simulink model "ControlDataSSM0709"  (R2023b)
settings: Solver=FixedStepAuto  StartTime=0.0  StopTime=inf  FixedStep=0.01  RelTol=1e-3
undefined symbols (not defined in the file): Down, Pull
libraries: simulink x39, speedgoatlib_IO691 x23, canmsglib x22, slrealtimeutilitieslib x1, slrealtimeiplib x1
(part 1 of 2)
settings Model: Creator=86188  LastModifiedBy=86188
settings SolverCC: ConcurrentTasks=on  PositivePriorityOrder=on
settings OptimizationCC: BlockReduction=off  OptimizeBlockIOStorage=off  BufferReuse=off
settings DebuggingCC: AlgebraicLoopMsg=none  TasksWithSamePriorityMsg=none
settings HardwareCC: ProdBitPerLong=64  ProdLongLongMode=on  ProdHWDeviceType=Intel->x86-64 (Linux 64)
settings RTWCC: Description=Simulink Real-Time  SystemTargetFile=slrealtime.tlc  TemplateMakefile=slrealtime_default_tmf  Toolchain=Simulink Real-Time Toolchain  BuildConfiguration=Faster Runs  CodeExecutionProfiling=on  TargetLang=C++

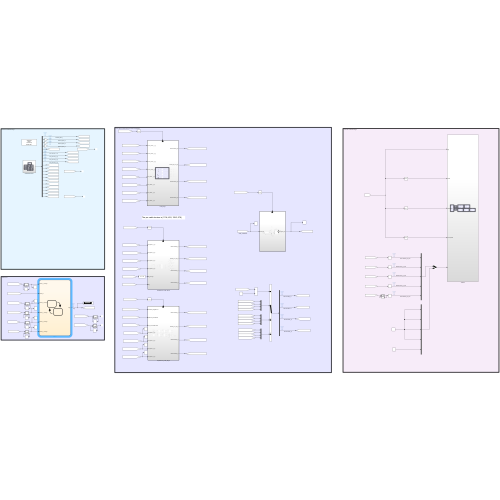
[thumbnail: Simulink's stored preview of the top-level diagram]
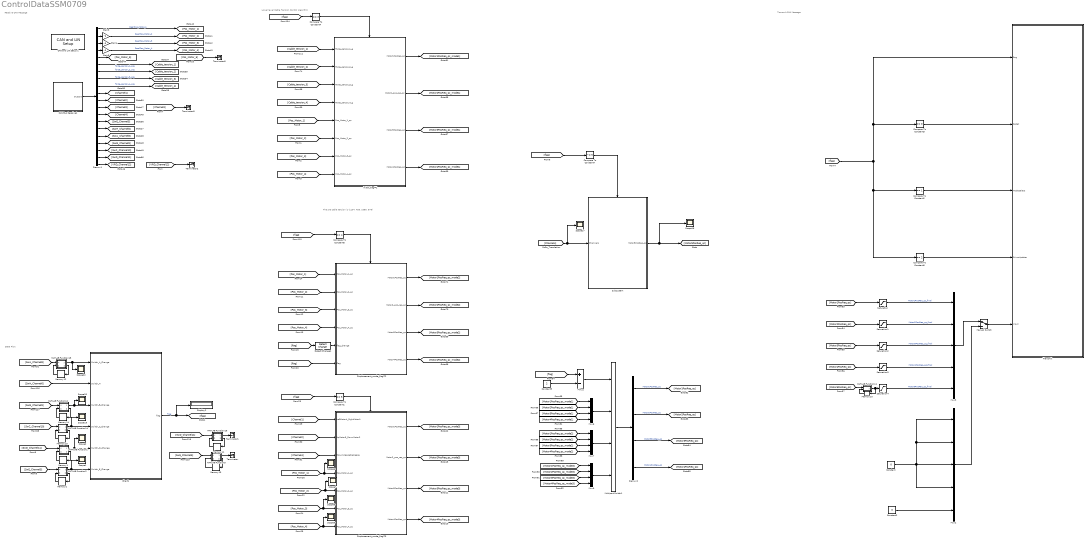
== system ControlDataSSM0709 ==
  note: Transmit CAN Message
  note: Receive CAN Message
  note: Lower level Cable Tension Control Algorithm
  note: The pre cable tension is (1104, 455, 1080, 978)
  note: Stata Flow
  CAN Bus Receive1 : Subsystem
  CAN and LIN Setup 1 : speedgoatlib_IO691/CAN and LIN Setup   moduleInitValues="[691    1    1   -1   -1]"  id=1  moduleType=IO691  pciSlot=-1  canChn1=CAN (HS)  canChn2=CAN (HS)  canChn3=Disabled  canChn4=Disabled  linChn1=Disabled  linChn2=Disabled  canInitStructArray=[]  canTermStructArray=[]  gpioChnx=Disabled  canChn1InitValues="[2   2   8   1  16   3  19   2   2   5   2   0]"  arbBdrChn1=500 kBaud  clockDividerChn1=Enable  arbManBdrChn1=[8,1,16,3]  fdBdrChn1=5.0 MBaud  fdManBdrChn1=[2,2,5,2]  termResistor1=off  canChn2InitValues="[2   2   8   1  16   3  19   2   2   5   2   0]"  arbBdrChn2=500 kBaud  clockDividerChn2=Enable  arbManBdrChn2=[8,1,16,3]  fdBdrChn2=5.0 MBaud  fdManBdrChn2=[2,2,5,2]  termResistor2=off  canChn3InitValues="[1   0   2   8  31   8  19   2   2   5   2   0]"  arbBdrChn3=1.0 MBaud  clockDividerChn3=Enable  arbManBdrChn3=[2,8,31,8]  fdBdrChn3=5.0 MBaud  fdManBdrChn3=[2,2,5,2]  termResistor3=off  canChn4InitValues="[1   0   2   8  31   8  19   2   2   5   2   0]"  arbBdrChn4=1.0 MBaud  clockDividerChn4=Enable  arbManBdrChn4=[2,8,31,8]  fdBdrChn4=5.0 MBaud  fdManBdrChn4=[2,2,5,2]  termResistor4=off  linChn1InitValues="[0  9600]"  linBtrChn1=9600  linChn2InitValues="[0  9600]"  linBtrChn2=9600  doInitTermStruct="[0  5  0  0  0]"  parDoChannels=[1 2]  parDoVoltage=5  parDoInitValues=0  parDoReset=1  parNumOfDoS=0  parDiChannels=[3 4]  parDiVoltage=5  parDiPull=Pull-Down
      settings: SourceProductName=Simulink Real-Time: Speedgoat I/O Blockset
  Chart1 : Stateflow chart  TreatAsAtomicUnit=on
  Compare To Constant1 : simulink/Logic and Bit Operations/Compare To Constant  relop===  const=5  OutDataTypeStr=boolean
  Compare To Constant2 : simulink/Logic and Bit Operations/Compare To Constant  relop===  const=1  OutDataTypeStr=boolean
  Compare To Constant3 : simulink/Logic and Bit Operations/Compare To Constant  relop===  const=0  OutDataTypeStr=boolean
  Compare To Constant4 : simulink/Logic and Bit Operations/Compare To Constant  relop===  const=3  OutDataTypeStr=boolean
  Compare To Constant5 : simulink/Logic and Bit Operations/Compare To Constant  relop===  const=2  OutDataTypeStr=boolean
  Compare To Constant6 : simulink/Logic and Bit Operations/Compare To Constant  relop===  const=4  OutDataTypeStr=boolean
  Compare To Constant7 : simulink/Logic and Bit Operations/Compare To Constant  relop=~=  const=5  OutDataTypeStr=boolean
  Constant : Constant  Value=0
  Constant2 : Constant  Value=0
  Constant3 : Constant  Value=2
  Demux1 : Demux  Outputs=20
  Demux2 : Demux
  Detect Change1 : simulink/Logic and Bit Operations/Detect Change  vinit=0  OutDataTypeStr=boolean
  Displacement_mode_flag=2 : Subsystem
  Displacement_mode_flag=3 : Subsystem
  Display2 : Display
  Gain3 : Gain  Gain=-1
  Gain4 : Gain  Gain=-1
  Gain5 : Gain  Gain=-1
  Initial_flag=1 : Subsystem
  MATLAB Function1 : MATLAB Function  TreatAsAtomicUnit=on
  MATLAB Function11 : MATLAB Function  TreatAsAtomicUnit=on
  MATLAB Function12 : MATLAB Function  TreatAsAtomicUnit=on
  MATLAB Function14 : MATLAB Function  TreatAsAtomicUnit=on
  MATLAB Function15 : MATLAB Function  TreatAsAtomicUnit=on
  MATLAB Function16 : MATLAB Function  TreatAsAtomicUnit=on
  MATLAB Function2 : MATLAB Function  TreatAsAtomicUnit=on
  MATLAB Function5 : MATLAB Function  TreatAsAtomicUnit=on
  Manual Switch : ManualSwitch
  Memory{1..2,10..15} (8 alike) : Memory
  Minus : Sum  Inputs=+-
  Multiport Switch1 : MultiPortSwitch  SaturateOnIntegerOverflow=off  InputSameDT=off
  Mux2 : Mux  Inputs=5
  Mux3 : Mux  Inputs=5
  Mux6 : Mux
  Mux7 : Mux
  Mux9 : Mux
  Saturation{,1..3} (4 alike) : Saturate  UpperLimit=6000  LowerLimit=-6000
  Saturation4 : Saturate  UpperLimit=8000  LowerLimit=-8000
  Scope{1..2,6..9,16..17,19..20,22} (11 alike) : Scope
  Subsystem : Subsystem
  Terminator{,1..3,5} (5 alike) : Terminator
  Transmit : Subsystem
  wires:
  Multiport Switch1/1 -> Demux2/1
  [Motor1PosReq_qc_mode2] -> Mux7/1
  Manual Switch/1 -> Transmit/5(Input)
  [Motor2PosReq_qc_mode3] -> Mux9/2
  [Motor3PosReq_qc_mode2] -> Mux7/3
  [Motor2PosReq_qc_mode1] -> Mux6/2
  [Motor4PosReq_qc_mode1] -> Mux6/4
  Initial_flag=1/2(Motor2_pos_req_qc) -> [Motor2PosReq_qc_mode1]
  Mux9/1 -> Multiport Switch1/4
  Initial_flag=1/3(Motor3PosReq_qc) -> [Motor3PosReq_qc_mode1]
  [Motor4PosReq_qc_mode3] -> Mux9/4
  [Motor1PosReq_qc_mode3] -> Mux9/1
  [Motor3PosReq_qc_mode3] -> Mux9/3
  [flag] -> Compare To Constant4/1
  Displacement_mode_flag=2/3(Motor3PosReq_qc) -> [Motor3PosReq_qc_mode2]
  Displacement_mode_flag=2/2(Motor2_pos_req_qc) -> [Motor2PosReq_qc_mode2]
  Displacement_mode_flag=2/4(Motor4PosReq_qc) -> [Motor4PosReq_qc_mode2]
  [Motor3PosReq_qc] -> Saturation2/1
  [flag] -> Transmit/1(flag), Compare To Constant3/1, Compare To Constant5/1, Compare To Constant2/1
  [Motor1PosReq_qc_mode1] -> Mux6/1
  Mux7/1 -> Multiport Switch1/3
  Displacement_mode_flag=2/1(Motor1PosReq_qc) -> [Motor1PosReq_qc_mode2]
  Initial_flag=1/4(Motor4PosReq_qc) -> [Motor4PosReq_qc_mode1]
  [Cable_tension_4] -> Initial_flag=1/4(Force_sensor_4_g)
  Compare To Constant4/1 -> Initial_flag=1/Enable
  [flag] -> Compare To Constant6/1
  Mux6/1 -> Multiport Switch1/2
  [Cable_tension_3] -> Initial_flag=1/3(Force_sensor_3_g)
  [Motor3PosReq_qc_mode1] -> Mux6/3
  Mux2/1 -> Manual Switch/2
  [Motor4PosReq_qc_mode2] -> Mux7/4
  [Motor2PosReq_qc_mode2] -> Mux7/2
  Compare To Constant6/1 -> Displacement_mode_flag=2/Enable
  [Cable_tension_2] -> Initial_flag=1/2(Force_sensor_2_g)
  [Cable_tension_1] -> Initial_flag=1/1(Force_sensor_1_g)
  Initial_flag=1/1(Motor1PosReq_qc) -> [Motor1PosReq_qc_mode1]
  Compare To Constant3/1 -> Transmit/2(ReSet)
  [Pos_Motor_2] -> Displacement_mode_flag=2/2(Pos_Motor_2_qc)
  [Pos_Motor_1] -> Displacement_mode_flag=2/1(Pos_Motor_1_qc)
  [Pos_Motor_3] -> Displacement_mode_flag=2/3(Pos_Motor_3_qc)
  [Pos_Motor_4] -> Displacement_mode_flag=2/4(Pos_Motor_4_qc)
  [flag] -> Detect Change1/1
  [flag] -> Displacement_mode_flag=2/6(flag)
  Detect Change1/1 -> Displacement_mode_flag=2/5(flag_change)
  [Pos_Motor_1] -> Scope6/1, Displacement_mode_flag=3/4(Pos_Motor_1_qc)
  [Pos_Motor_4] -> Scope9/1, Displacement_mode_flag=3/7(Pos_Motor_4_qc)
  [flag] -> Compare To Constant1/1
  [Pos_Motor_3] -> Scope8/1, Displacement_mode_flag=3/6(Pos_Motor_3_qc)
  [Pos_Motor_2] -> Scope7/1, Displacement_mode_flag=3/5(Pos_Motor_2_qc)
  [Channel2] -> Displacement_mode_flag=3/2(UpMotor3_DownMotor2)
  [Channel1] -> Displacement_mode_flag=3/1(LeftMotor4_RightMotor1)
  Compare To Constant1/1 -> Displacement_mode_flag=3/Enable
  Displacement_mode_flag=3/1(Motor1PosReq_qc) -> [Motor1PosReq_qc_mode3]
  Displacement_mode_flag=3/3(Motor3PosReq_qc) -> [Motor3PosReq_qc_mode3]
  Displacement_mode_flag=3/4(Motor4PosReq_qc) -> [Motor4PosReq_qc_mode3]
  Displacement_mode_flag=3/2(Motor2_pos_req_qc) -> [Motor2PosReq_qc_mode3]
  [Channel4] -> Displacement_mode_flag=3/3(Pos_IncreaseDecrease)
  Saturation4/1 -> Mux3/5  "Motor5PosReq_qc_final"
  Mux3/1 -> Manual Switch/1
  Saturation3/1 -> Mux3/4  "Motor4PosReq_qc_final"
  Saturation/1 -> Mux3/1  "Motor1PosReq_qc_final"
  Saturation1/1 -> Mux3/2  "Motor2PosReq_qc_final"
  Saturation2/1 -> Mux3/3  "Motor3PosReq_qc_final"
  [Motor2PosReq_qc] -> Saturation1/1
  [Motor4PosReq_qc] -> Saturation3/1
  MATLAB Function11/1(y) -> Memory10/1, Saturation4/1
  Memory10/1 -> MATLAB Function11/2(u_last)
  Demux2/1 -> [Motor1PosReq_qc]  "Motor1PosReq_qc"
  Demux2/2 -> [Motor2PosReq_qc]  "Motor2PosReq_qc"
  Demux2/3 -> [Motor3PosReq_qc]  "Motor3PosReq_qc"
  Demux2/4 -> [Motor4PosReq_qc]  "Motor4PosReq_qc"
  [Motor5PosReq_qc] -> MATLAB Function11/1(u)
  [Channel4] -> Subsystem/1(Channel4), Scope17/1
  Subsystem/1(Motor5PosReq_qc) -> Scope16/1, [Motor5PosReq_qc]
  Constant/1 -> Mux2/4, Mux2/1, Mux2/2, Mux2/3
  Constant2/1 -> Mux2/5
  Demux1/16 -> [SwA_Channel8]
  Demux1/18 -> [SwC_Channel10]
  Demux1/14 -> [SwE_Channel5]
  Demux1/9 -> [Cable_tension_4]  "force_sensor_4_org"
  CAN Bus Receive1/1(Outport) -> Demux1/1
  Demux1/19 -> [SwD_Channel11]
  Demux1/6 -> [Cable_tension_1]  "force_sensor_1_org"
  Demux1/1 -> [Pos_Motor_1]  "RealPos_Motor_1"
  Demux1/12 -> [Channel3]
  Demux1/3 -> Gain4/1
  Demux1/5 -> [Pos_Motor_5]
  Demux1/11 -> [Channel2]
  Demux1/8 -> [Cable_tension_3]  "force_sensor_3_org"
  Demux1/20 -> [VRD_Channel12]
  Gain4/1 -> [Pos_Motor_3]  "RealPos_Motor_3"
  Demux1/13 -> [Channel4]
  Demux1/15 -> [SwH_Channel6]
  Demux1/7 -> [Cable_tension_2]  "force_sensor_2_org"
  Gain5/1 -> [Pos_Motor_4]  "RealPos_Motor_4"
  Demux1/10 -> [Channel1]
  Demux1/4 -> Gain5/1
  Demux1/2 -> Gain3/1
  Gain3/1 -> [Pos_Motor_2]  "RealPos_Motor_2"
  Demux1/17 -> [SwB_Channel9]
  [SwB_Channel9] -> MATLAB Function12/1(u)
  Memory14/1 -> MATLAB Function12/2(u_last)
  MATLAB Function16/2(u_out) -> Memory11/1
  MATLAB Function14/2(u_out) -> Memory15/1
  MATLAB Function15/2(u_out) -> Memory12/1
  MATLAB Function15/1(y) -> Scope22/1, Chart1/1(Switch_A_Change)
  MATLAB Function14/1(y) -> Scope19/1, Chart1/4(Switch_C_Change)
  [SwA_Channel8] -> MATLAB Function15/1(u)
  [SwE_Channel5] -> MATLAB Function5/1(u)
  MATLAB Function5/2(u_out) -> Memory13/1
  Memory12/1 -> MATLAB Function15/2(u_last)
  Chart1/1(flag) -> Display2/1, [flag]  "flag"
  Memory11/1 -> MATLAB Function16/2(u_last)
  [SwH_Channel6] -> Chart1/2(Switch_H)
  MATLAB Function12/2(u_out) -> Memory14/1
  [SwD_Channel11] -> MATLAB Function16/1(u)
  MATLAB Function12/1(y) -> Scope20/1, Chart1/3(Switch_B_Change)
  Memory13/1 -> MATLAB Function5/2(u_last)
  Memory15/1 -> MATLAB Function14/2(u_last)
  [SwC_Channel10] -> MATLAB Function14/1(u)
  MATLAB Function5/1(y) -> Terminator/1
  MATLAB Function16/1(y) -> Terminator1/1
  [Pos_Motor_1] -> Initial_flag=1/5(Pos_Motor_1_qc)
  [Pos_Motor_2] -> Initial_flag=1/6(Pos_Motor_2_qc)
  [Pos_Motor_3] -> Initial_flag=1/7(Pos_Motor_3_qc)
  [Pos_Motor_4] -> Initial_flag=1/8(Pos_Motor_4_qc)
  [SwD_Channel11] -> MATLAB Function1/1(u)
  Memory1/1 -> MATLAB Function1/2(u_last)
  [SwE_Channel5] -> MATLAB Function2/1(u)
  MATLAB Function1/1(y) -> Chart1/5(Switch_D_Change), Scope2/1
  MATLAB Function2/2(u_out) -> Memory2/1
  Memory2/1 -> MATLAB Function2/2(u_last)
  MATLAB Function2/1(y) -> Chart1/6(Switch_E_Change), Scope1/1
  MATLAB Function1/2(u_out) -> Memory1/1
  Compare To Constant2/1 -> Transmit/3(ModeSelect)
  Compare To Constant5/1 -> Transmit/4(DriverUpdate)
  Minus/1 -> Multiport Switch1/1
  [flag] -> Minus/1
  Constant3/1 -> Minus/2
  [flag] -> Compare To Constant7/1
  Compare To Constant7/1 -> Subsystem/Enable
  [VRD_Channel12] -> Terminator2/1
  [Channel3] -> Terminator3/1
  [Pos_Motor_5] -> Terminator5/1
  [Motor1PosReq_qc] -> Saturation/1

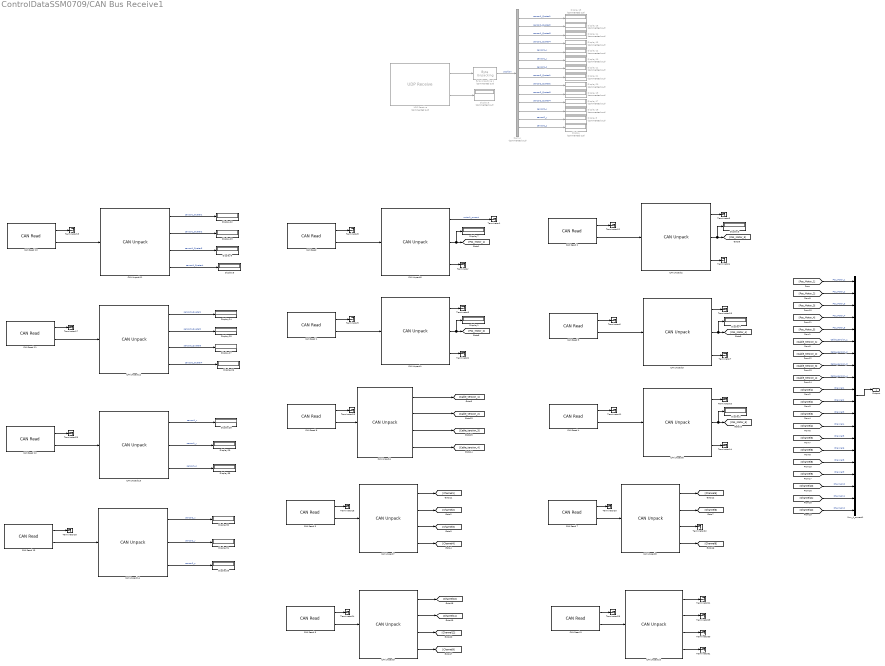
== system ControlDataSSM0709/CAN Bus Receive1 ==
  Byte Unpacking 1 : slrealtimeutilitieslib/Byte Unpacking  Commented=on  MaskUnpackedDataTypes={'double'}  MaskUnpackedDataSizes={[14]}  MaskAlignment=1
  "CAN Read " : speedgoatlib_IO691/CAN Read   moduleType=IO691  id=1  channel=1  canType=CAN (HS)  messageType=CAN (HS)  useBusOut=off  HasMulRead=Specify by IDs  MsgIDlist=[27]  isEFF=off  LabelInHex=on  enableInput=off  initValues=[691 1 0.01 0 1 1 0 0 2 0 1 27]  ts=0.01
      settings: SourceProductName=Simulink Real-Time: Speedgoat I/O Blockset
  CAN Read 1 : speedgoatlib_IO691/CAN Read   moduleType=IO691  id=1  channel=1  canType=CAN (HS)  messageType=CAN (HS)  useBusOut=off  HasMulRead=Specify by IDs  MsgIDlist=[43]  isEFF=off  LabelInHex=on  enableInput=off  initValues=[691 1 0.01 0 1 1 0 0 2 0 1 43]  ts=0.01
      settings: SourceProductName=Simulink Real-Time: Speedgoat I/O Blockset
  CAN Read 10 : speedgoatlib_IO691/CAN Read   moduleType=IO691  id=1  channel=1  canType=CAN (HS)  messageType=CAN (HS)  useBusOut=off  HasMulRead=Specify by IDs  MsgIDlist=[113]  isEFF=off  LabelInHex=on  enableInput=off  initValues=[691 1 0.01 0 1 1 0 0 2 0 1 113]  ts=0.01
      settings: SourceProductName=Simulink Real-Time: Speedgoat I/O Blockset
  CAN Read 11 : speedgoatlib_IO691/CAN Read   moduleType=IO691  id=1  channel=1  canType=CAN (HS)  messageType=CAN (HS)  useBusOut=off  HasMulRead=Specify by IDs  MsgIDlist=[115]  isEFF=off  LabelInHex=on  enableInput=off  initValues=[691 1 0.01 0 1 1 0 0 2 0 1 115]  ts=0.01
      settings: SourceProductName=Simulink Real-Time: Speedgoat I/O Blockset
  CAN Read 12 : speedgoatlib_IO691/CAN Read   moduleType=IO691  id=1  channel=1  canType=CAN (HS)  messageType=CAN (HS)  useBusOut=off  HasMulRead=Specify by IDs  MsgIDlist=[114]  isEFF=off  LabelInHex=on  enableInput=off  initValues=[691 1 0.01 0 1 1 0 0 2 0 1 114]  ts=0.01
      settings: SourceProductName=Simulink Real-Time: Speedgoat I/O Blockset
  CAN Read 13 : speedgoatlib_IO691/CAN Read   moduleType=IO691  id=1  channel=1  canType=CAN (HS)  messageType=CAN (HS)  useBusOut=off  HasMulRead=Specify by IDs  MsgIDlist=[116]  isEFF=off  LabelInHex=on  enableInput=off  initValues=[691 1 0.01 0 1 1 0 0 2 0 1 116]  ts=0.01
      settings: SourceProductName=Simulink Real-Time: Speedgoat I/O Blockset
  CAN Read 2 : speedgoatlib_IO691/CAN Read   moduleType=IO691  id=1  channel=1  canType=CAN (HS)  messageType=CAN (HS)  useBusOut=off  HasMulRead=Specify by IDs  MsgIDlist=[59]  isEFF=off  LabelInHex=on  enableInput=off  initValues=[691 1 0.01 0 1 1 0 0 2 0 1 59]  ts=0.01
      settings: SourceProductName=Simulink Real-Time: Speedgoat I/O Blockset
  CAN Read 3 : speedgoatlib_IO691/CAN Read   moduleType=IO691  id=1  channel=1  canType=CAN (HS)  messageType=CAN (HS)  useBusOut=off  HasMulRead=Specify by IDs  MsgIDlist=[75]  isEFF=off  LabelInHex=on  enableInput=off  initValues=[691 1 0.01 0 1 1 0 0 2 0 1 75]  ts=0.01
      settings: SourceProductName=Simulink Real-Time: Speedgoat I/O Blockset
  CAN Read 4 : speedgoatlib_IO691/CAN Read   moduleType=IO691  id=1  channel=1  canType=CAN (HS)  messageType=CAN (HS)  useBusOut=off  HasMulRead=Specify by IDs  MsgIDlist=[91]  isEFF=off  LabelInHex=on  enableInput=off  initValues=[691 1 0.01 0 1 1 0 0 2 0 1 91]  ts=0.01
      settings: SourceProductName=Simulink Real-Time: Speedgoat I/O Blockset
  CAN Read 5 : speedgoatlib_IO691/CAN Read   moduleType=IO691  id=1  channel=1  canType=CAN (HS)  messageType=CAN (HS)  useBusOut=off  HasMulRead=Specify by IDs  MsgIDlist=[391]  isEFF=off  LabelInHex=on  enableInput=off  initValues=[691 1 0.01 0 1 1 0 0 2 0 1 391]  ts=0.01
      settings: SourceProductName=Simulink Real-Time: Speedgoat I/O Blockset
  CAN Read 6 : speedgoatlib_IO691/CAN Read   moduleType=IO691  id=1  channel=1  canType=CAN (HS)  messageType=CAN (HS)  useBusOut=off  HasMulRead=Specify by IDs  MsgIDlist=[529024]  isEFF=on  LabelInHex=on  enableInput=off  initValues=[691 1 0.01 0 1 1 0 0 2 1 1 529024]  ts=0.01
      settings: SourceProductName=Simulink Real-Time: Speedgoat I/O Blockset
  CAN Read 7 : speedgoatlib_IO691/CAN Read   moduleType=IO691  id=1  channel=1  canType=CAN (HS)  messageType=CAN (HS)  useBusOut=off  HasMulRead=Specify by IDs  MsgIDlist=[392]  isEFF=off  LabelInHex=on  enableInput=off  initValues=[691 1 0.01 0 1 1 0 0 2 0 1 392]  ts=0.01
      settings: SourceProductName=Simulink Real-Time: Speedgoat I/O Blockset
  CAN Read 8 : speedgoatlib_IO691/CAN Read   moduleType=IO691  id=1  channel=1  canType=CAN (HS)  messageType=CAN (HS)  useBusOut=off  HasMulRead=Specify by IDs  MsgIDlist=[393]  isEFF=off  LabelInHex=on  enableInput=off  initValues=[691 1 0.01 0 1 1 0 0 2 0 1 393]  ts=0.01
      settings: SourceProductName=Simulink Real-Time: Speedgoat I/O Blockset
  CAN Read 9 : speedgoatlib_IO691/CAN Read   moduleType=IO691  id=1  channel=1  canType=CAN (HS)  messageType=CAN (HS)  useBusOut=off  HasMulRead=Specify by IDs  MsgIDlist=[394]  isEFF=off  LabelInHex=on  enableInput=off  initValues=[691 1 0.01 0 1 1 0 0 2 0 1 394]  ts=0.01
      settings: SourceProductName=Simulink Real-Time: Speedgoat I/O Blockset
  CAN Unpack1 : canmsglib/CAN Unpack  CANdbFile=E:\OneDrive\OneDrive - The Chinese University of Hong Kong\文档\Research\SRIL\12nd\Experiment\Simulink\RoboModule0729.dbc  MsgList=Feedback_curvelpos_Dv2  MsgName=Feedback_curvelpos_Dv2  MsgIDType=Standard (11-bit identifier)  MsgIdentifier=43  MsgLength=8  SignalInfo={'real_current','8','16','BE','signed','Standard','0','1','0','-Inf','Inf';'real_position','56','32','BE','signed','Standard','0','1','0','-Inf','Inf';'real_velocity','24','16','BE','signed','Standard','0','1','0','-Inf','Inf'}  IDPort=off  TimestampPort=off  ErrorPort=off  RemotePort=off  LengthPort=off  StatusPort=off  ApplyMinMax=off
      settings: DataFormat=CANdb specified signals
  CAN Unpack10 : canmsglib/CAN Unpack  CANdbFile=E:\OneDrive\OneDrive - The Chinese University of Hong Kong\文档\Research\SRIL\12nd\Experiment\Simulink\RoboModule0729.dbc  MsgList=RadioLink_4  MsgName=RadioLink_4  MsgIDType=Standard (11-bit identifier)  MsgIdentifier=394  MsgLength=8  SignalInfo={'Channel13','8','16','BE','unsigned','Standard','0','1','0','-Inf','Inf';'Channel14','24','16','BE','unsigned','Standard','0','1','0','-Inf','Inf';'Channel15','40','16','BE','unsigned','Standard','0','1','0','-Inf','Inf';'Channel16','56','16','BE','unsigned','Standard','0','1','0','-Inf','Inf'}  IDPort=off  TimestampPort=off  ErrorPort=off  RemotePort=off  LengthPort=off  StatusPort=off  ApplyMinMax=off
      settings: DataFormat=CANdb specified signals
  CAN Unpack11 : canmsglib/CAN Unpack  CANdbFile=E:\Research\SRIL\14th\TroRevision\datacollection\ControlEmbedding\RoboModule0729.dbc  MsgList=Sensor1Quater  MsgName=Sensor1Quater  MsgIDType=Standard (11-bit identifier)  MsgIdentifier=113  MsgLength=8  SignalInfo={'Quater1','8','16','BE','signed','Standard','0','0.0001','0','-3.2768','3.2767';'Quater2','24','16','BE','signed','Standard','0','0.0001','0','-3.2768','3.2767';'Quater3','40','16','BE','signed','Standard','0','0.0001','0','-Inf','Inf';'Quater4','56','16','BE','signed','Standard','0','0.0001','0','-3.2768','3.2767'}  IDPort=off  TimestampPort=off  ErrorPort=off  RemotePort=off  LengthPort=off  StatusPort=off  ApplyMinMax=off
      settings: DataFormat=CANdb specified signals
  CAN Unpack12 : canmsglib/CAN Unpack  CANdbFile=E:\Research\SRIL\14th\TroRevision\datacollection\ControlEmbedding\RoboModule0729.dbc  MsgList=Sensor2Quater  MsgName=Sensor2Quater  MsgIDType=Standard (11-bit identifier)  MsgIdentifier=115  MsgLength=8  SignalInfo={'Quater1','8','16','BE','signed','Standard','0','0.0001','0','-3.2768','3.2767';'Quater2','24','16','BE','signed','Standard','0','0.0001','0','-3.2768','3.2767';'Quater3','40','16','BE','signed','Standard','0','0.0001','0','-3.2768','3.2767';'Quater4','56','16','BE','signed','Standard','0','0.0001','0','-3.2768','3.2767'}  IDPort=off  TimestampPort=off  ErrorPort=off  RemotePort=off  LengthPort=off  StatusPort=off  ApplyMinMax=off
      settings: DataFormat=CANdb specified signals
  CAN Unpack13 : canmsglib/CAN Unpack  CANdbFile=E:\Research\SRIL\14th\TroRevision\datacollection\ControlEmbedding\RoboModule0729.dbc  MsgList=Sensor1Pos  MsgName=Sensor1Pos  MsgIDType=Standard (11-bit identifier)  MsgIdentifier=114  MsgLength=8  SignalInfo={'PosX','8','16','BE','signed','Standard','0','0.01','0','-Inf','Inf';'PosY','24','16','BE','signed','Standard','0','0.01','0','-Inf','Inf';'PosZ','40','16','BE','signed','Standard','0','0.01','0','-Inf','Inf'}  IDPort=off  TimestampPort=off  ErrorPort=off  RemotePort=off  LengthPort=off  StatusPort=off  ApplyMinMax=off
      settings: DataFormat=CANdb specified signals
  CAN Unpack14 : canmsglib/CAN Unpack  CANdbFile=E:\Research\SRIL\14th\TroRevision\datacollection\ControlEmbedding\RoboModule0729.dbc  MsgList=Sensor2Pos  MsgName=Sensor2Pos  MsgIDType=Standard (11-bit identifier)  MsgIdentifier=116  MsgLength=8  SignalInfo={'PosX','8','16','BE','signed','Standard','0','0.01','0','-327.68','327.67';'PosY','24','16','BE','signed','Standard','0','0.01','0','-327.68','327.67';'PosZ','40','16','BE','signed','Standard','0','0.01','0','-327.68','327.67'}  IDPort=off  TimestampPort=off  ErrorPort=off  RemotePort=off  LengthPort=off  StatusPort=off  ApplyMinMax=off
      settings: DataFormat=CANdb specified signals
  CAN Unpack2 : canmsglib/CAN Unpack  CANdbFile=E:\OneDrive\OneDrive - The Chinese University of Hong Kong\文档\Research\SRIL\12nd\Experiment\Simulink\RoboModule0729.dbc  MsgList=Feedback_curvelpos_Dv3  MsgName=Feedback_curvelpos_Dv3  MsgIDType=Standard (11-bit identifier)  MsgIdentifier=59  MsgLength=8  SignalInfo={'real_current','8','16','BE','signed','Standard','0','1','0','-Inf','Inf';'real_position','56','32','BE','signed','Standard','0','1','0','-Inf','Inf';'real_velocity','24','16','BE','signed','Standard','0','1','0','-Inf','Inf'}  IDPort=off  TimestampPort=off  ErrorPort=off  RemotePort=off  LengthPort=off  StatusPort=off  ApplyMinMax=off
      settings: DataFormat=CANdb specified signals
  CAN Unpack3 : canmsglib/CAN Unpack  CANdbFile=E:\OneDrive\OneDrive - The Chinese University of Hong Kong\文档\Research\SRIL\12nd\Experiment\Simulink\RoboModule0729.dbc  MsgList=Feedback_curvelpos_Dr4  MsgName=Feedback_curvelpos_Dr4  MsgIDType=Standard (11-bit identifier)  MsgIdentifier=75  MsgLength=8  SignalInfo={'real_current','8','16','BE','signed','Standard','0','1','0','-Inf','Inf';'real_position','56','32','BE','signed','Standard','0','1','0','-Inf','Inf';'real_velocity','24','16','BE','signed','Standard','0','1','0','-Inf','Inf'}  IDPort=off  TimestampPort=off  ErrorPort=off  RemotePort=off  LengthPort=off  StatusPort=off  ApplyMinMax=off
      settings: DataFormat=CANdb specified signals
  CAN Unpack4 : canmsglib/CAN Unpack  CANdbFile=E:\OneDrive\OneDrive - The Chinese University of Hong Kong\文档\Research\SRIL\12nd\Experiment\Simulink\RoboModule0729.dbc  MsgList=Cable_tension  MsgName=Cable_tension  MsgIDType=Extended (29-bit identifier)  MsgIdentifier=529024  MsgLength=8  SignalInfo={'Force_sensor_1','8','16','BE','unsigned','Standard','0','1','0','-Inf','Inf';'Force_sensor_2','24','16','BE','unsigned','Standard','0','1','0','-Inf','Inf';'Force_sensor_3','40','16','BE','unsigned','Standard','0','1','0','-Inf','Inf';'Force_sensor_4','56','16','BE','unsigned','Standard','0','1','0','-Inf','Inf'}  IDPort=off  TimestampPort=off  ErrorPort=off  RemotePort=off  LengthPort=off  StatusPort=off  ApplyMinMax=off
      settings: DataFormat=CANdb specified signals
  CAN Unpack5 : canmsglib/CAN Unpack  CANdbFile=E:\OneDrive\OneDrive - The Chinese University of Hong Kong\文档\Research\SRIL\12nd\Experiment\Simulink\RoboModule0729.dbc  MsgList=Feedback_curvelpos_Dv1  MsgName=Feedback_curvelpos_Dv1  MsgIDType=Standard (11-bit identifier)  MsgIdentifier=27  MsgLength=8  SignalInfo={'real_current','8','16','BE','signed','Standard','0','1','0','-Inf','Inf';'real_position','56','32','BE','signed','Standard','0','1','0','-Inf','Inf';'real_velocity','24','16','BE','signed','Standard','0','1','0','-Inf','Inf'}  IDPort=off  TimestampPort=off  ErrorPort=off  RemotePort=off  LengthPort=off  StatusPort=off  ApplyMinMax=off
      settings: DataFormat=CANdb specified signals
  CAN Unpack6 : canmsglib/CAN Unpack  CANdbFile=E:\OneDrive\OneDrive - The Chinese University of Hong Kong\文档\Research\SRIL\12nd\Experiment\Simulink\RoboModule0729.dbc  MsgList=Feedback_curvelpos_Dr5  MsgName=Feedback_curvelpos_Dr5  MsgIDType=Standard (11-bit identifier)  MsgIdentifier=91  MsgLength=8  SignalInfo={'real_current','8','16','BE','signed','Standard','0','1','0','-Inf','Inf';'real_position','56','32','BE','signed','Standard','0','1','0','-Inf','Inf';'real_velocity','24','16','BE','signed','Standard','0','1','0','-Inf','Inf'}  IDPort=off  TimestampPort=off  ErrorPort=off  RemotePort=off  LengthPort=off  StatusPort=off  ApplyMinMax=off
      settings: DataFormat=CANdb specified signals
  CAN Unpack7 : canmsglib/CAN Unpack  CANdbFile=E:\OneDrive\OneDrive - The Chinese University of Hong Kong\文档\Research\SRIL\12nd\Experiment\Simulink\RoboModule0729.dbc  MsgList=RadioLink_1  MsgName=RadioLink_1  MsgIDType=Standard (11-bit identifier)  MsgIdentifier=391  MsgLength=8  SignalInfo={'Channel1','8','16','BE','unsigned','Standard','0','1','0','-Inf','Inf';'Channel2','24','16','BE','unsigned','Standard','0','1','0','-Inf','Inf';'Channel3','40','16','BE','unsigned','Standard','0','1','0','-Inf','Inf';'Channel4','56','16','BE','unsigned','Standard','0','1','0','-Inf','Inf'}  IDPort=off  TimestampPort=off  ErrorPort=off  RemotePort=off  LengthPort=off  StatusPort=off  ApplyMinMax=off
      settings: DataFormat=CANdb specified signals
  CAN Unpack8 : canmsglib/CAN Unpack  CANdbFile=E:\OneDrive\OneDrive - The Chinese University of Hong Kong\文档\Research\SRIL\12nd\Experiment\Simulink\RoboModule0729.dbc  MsgList=RadioLink_2  MsgName=RadioLink_2  MsgIDType=Standard (11-bit identifier)  MsgIdentifier=392  MsgLength=8  SignalInfo={'Channel5','8','16','BE','unsigned','Standard','0','1','0','-Inf','Inf';'Channel6','24','16','BE','unsigned','Standard','0','1','0','-Inf','Inf';'Channel7','40','16','BE','unsigned','Standard','0','1','0','-Inf','Inf';'Channel8','56','16','BE','unsigned','Standard','0','1','0','-Inf','Inf'}  IDPort=off  TimestampPort=off  ErrorPort=off  RemotePort=off  LengthPort=off  StatusPort=off  ApplyMinMax=off
      settings: DataFormat=CANdb specified signals
  CAN Unpack9 : canmsglib/CAN Unpack  CANdbFile=E:\Research\SRIL\12nd\Simulink\RoboModule0729.dbc  MsgList=RadioLink_3  MsgName=RadioLink_3  MsgIDType=Standard (11-bit identifier)  MsgIdentifier=393  MsgLength=8  SignalInfo={'Channel10','24','16','BE','unsigned','Standard','0','1','0','-Inf','Inf';'Channel11','40','16','BE','unsigned','Standard','0','1','0','-Inf','Inf';'Channel12','56','16','BE','unsigned','Standard','0','1','0','-Inf','Inf';'Channel9','8','16','BE','unsigned','Standard','0','1','0','-Inf','Inf'}  IDPort=off  TimestampPort=off  ErrorPort=off  RemotePort=off  LengthPort=off  StatusPort=off  ApplyMinMax=off
      settings: DataFormat=CANdb specified signals
  Demux : Demux  Commented=on  Outputs=14
  Display{,6,8,10..21} (15 alike) : Display  Commented=on
  Display{1..5,7,9,22..31,33,35} (19 alike) : Display
      Display1 settings: Format=hex (Stored Integer)
      Display2 settings: Format=hex (Stored Integer)
      Display3 settings: Format=hex (Stored Integer)
      Display4 settings: Format=hex (Stored Integer)
      Display7 settings: Format=hex (Stored Integer)
  Mux_4_current1 : Mux  Inputs=20
  Terminator{,1..24,28..31} (29 alike) : Terminator
  UDP Receive : slrealtimeiplib/UDP Receive  Commented=on  useHostTargetConn=off  ipAddress=30.30.30.1  localPort=8001  rcvWidth=112  rcvFmAny=on  fmAddress='10.10.10.10'  sampleTime=-1  enableMessage=off  maxPackets=1
  Outport : Outport
  wires:
  CAN Unpack5/3 -> Terminator/1
  CAN Unpack4/1 -> [Cable_tension_1]
  CAN Unpack5/1 -> Terminator1/1  "motor1_current"
  "CAN Read "/2 -> CAN Unpack5/1
  CAN Unpack4/2 -> [Cable_tension_2]
  CAN Unpack5/2 -> Display7/1, [Pos_Motor_1]
  "CAN Read "/1 -> Terminator8/1
  CAN Read 1/2 -> CAN Unpack1/1
  CAN Read 1/1 -> Terminator9/1
  CAN Unpack1/2 -> Display1/1, [Pos_Motor_2]
  CAN Unpack1/3 -> Terminator2/1
  CAN Unpack1/1 -> Terminator3/1
  CAN Read 2/2 -> CAN Unpack2/1
  CAN Read 2/1 -> Terminator12/1
  CAN Unpack2/3 -> Terminator4/1
  CAN Unpack2/2 -> Display3/1, [Pos_Motor_3]
  CAN Unpack2/1 -> Terminator5/1
  CAN Read 3/2 -> CAN Unpack3/1
  CAN Unpack3/3 -> Terminator7/1
  CAN Read 3/1 -> Terminator6/1
  CAN Unpack3/1 -> Terminator13/1
  CAN Unpack3/2 -> Display4/1, [Pos_Motor_4]
  CAN Unpack6/2 -> Display2/1, [Pos_Motor_5]
  CAN Read 4/2 -> CAN Unpack6/1
  CAN Unpack6/1 -> Terminator10/1
  CAN Read 4/1 -> Terminator11/1
  CAN Unpack6/3 -> Terminator14/1
  CAN Read 6/1 -> Terminator15/1
  CAN Read 6/2 -> CAN Unpack4/1
  CAN Read 5/1 -> Terminator16/1
  CAN Read 5/2 -> CAN Unpack7/1
  CAN Unpack7/1 -> [Channel1]
  CAN Unpack7/2 -> [Channel2]
  CAN Unpack7/3 -> [Channel3]
  CAN Unpack7/4 -> [Channel4]
  CAN Unpack8/4 -> [Channel8]
  CAN Read 7/1 -> Terminator20/1
  CAN Unpack8/1 -> [Channel5]
  CAN Unpack8/2 -> [Channel6]
  CAN Read 7/2 -> CAN Unpack8/1
  CAN Unpack8/3 -> Terminator22/1
  CAN Unpack9/3 -> [Channel12]
  CAN Unpack9/1 -> [Channel10]
  CAN Read 8/2 -> CAN Unpack9/1
  CAN Read 8/1 -> Terminator24/1
  CAN Unpack9/2 -> [Channel11]
  CAN Unpack9/4 -> [Channel9]
  CAN Unpack10/2 -> Terminator29/1
  CAN Read 9/1 -> Terminator28/1
  CAN Unpack10/4 -> Terminator31/1
  CAN Read 9/2 -> CAN Unpack10/1
  CAN Unpack10/3 -> Terminator30/1
  CAN Unpack10/1 -> Terminator21/1
  [Channel1] -> Mux_4_current1/10  "Channel1"
  [Channel2] -> Mux_4_current1/11  "Channel2"
  [Channel4] -> Mux_4_current1/13  "Channel4"
  [Channel3] -> Mux_4_current1/12  "Channel3"
  [Channel5] -> Mux_4_current1/14  "Channel5"
  [Channel6] -> Mux_4_current1/15  "Channel6"
  CAN Unpack4/4 -> [Cable_tension_4]
  CAN Unpack4/3 -> [Cable_tension_3]
  [Pos_Motor_1] -> Mux_4_current1/1  "Pos_Motor_1"
  Mux_4_current1/1 -> Outport/1
  [Pos_Motor_2] -> Mux_4_current1/2  "Pos_Motor_2"
  [Pos_Motor_3] -> Mux_4_current1/3  "Pos_Motor_3"
  [Pos_Motor_4] -> Mux_4_current1/4  "Pos_Motor_4"
  [Pos_Motor_5] -> Mux_4_current1/5  "Pos_Motor_5"
  [Cable_tension_1] -> Mux_4_current1/6  "Cable_tension_1"
  [Cable_tension_2] -> Mux_4_current1/7  "Cable_tension_2"
  [Cable_tension_3] -> Mux_4_current1/8  "Cable_tension_3"
  [Cable_tension_4] -> Mux_4_current1/9  "Cable_tension_4"
  [Channel8] -> Mux_4_current1/16  "Channel8"
  [Channel10] -> Mux_4_current1/18  "Channel10"
  [Channel9] -> Mux_4_current1/17  "Channel9"
  [Channel11] -> Mux_4_current1/19  "Channel11"
  [Channel12] -> Mux_4_current1/20  "Channel12"
  Demux/3 -> Display14/1  "sensor1_Quater3"
  UDP Receive/1 -> Byte Unpacking 1/1
  Byte Unpacking 1/1 -> Demux/1  "position"
  Demux/4 -> Display13/1  "sensor1_Quater4"
  Demux/6 -> Display10/1  "sensor1_y"
  Demux/12 -> Display18/1  "sensor2_x"
  Demux/9 -> Display20/1  "sensor2_Quater2"
  Demux/2 -> Display16/1  "sensor1_Quater2"
  Demux/1 -> Display15/1  "sensor1_Quater1"
  Demux/8 -> Display21/1  "sensor2_Quater1"
  Demux/5 -> Display12/1  "sensor1_x"
  Demux/7 -> Display11/1  "sensor1_z"
  Demux/13 -> Display8/1  "sensor2_y"
  Demux/11 -> Display17/1  "sensor2_Quater4"
  UDP Receive/2 -> Display6/1
  Demux/14 -> Display/1  "sensor2_z"
  Demux/10 -> Display19/1  "sensor2_Quater3"
  CAN Read 10/2 -> CAN Unpack11/1
  CAN Read 10/1 -> Terminator19/1
  CAN Unpack11/2 -> Display23/1  "sensor1_Quater2"
  CAN Unpack11/1 -> Display22/1  "sensor1_Quater1"
  CAN Unpack11/4 -> Display5/1  "sensor1_Quater4"
  CAN Unpack11/3 -> Display9/1  "sensor1_Quater3"
  CAN Read 11/2 -> CAN Unpack12/1
  CAN Unpack12/2 -> Display25/1  "sensor2_Quater2"
  CAN Read 11/1 -> Terminator17/1
  CAN Unpack12/1 -> Display24/1  "sensor2_Quater1"
  CAN Unpack12/4 -> Display26/1  "sensor2_Quater4"
  CAN Unpack12/3 -> Display27/1  "sensor2_Quater3"
  CAN Read 12/2 -> CAN Unpack13/1
  CAN Read 13/1 -> Terminator18/1
  CAN Unpack14/3 -> Display33/1  "sensor2_z"
  CAN Unpack14/1 -> Display30/1  "sensor2_x"
  CAN Read 13/2 -> CAN Unpack14/1
  CAN Unpack14/2 -> Display31/1  "sensor2_y"
  CAN Unpack13/2 -> Display29/1  "sensor1_y"
  CAN Read 12/1 -> Terminator23/1
  CAN Unpack13/1 -> Display28/1  "sensor1_x"
  CAN Unpack13/3 -> Display35/1  "sensor1_z"

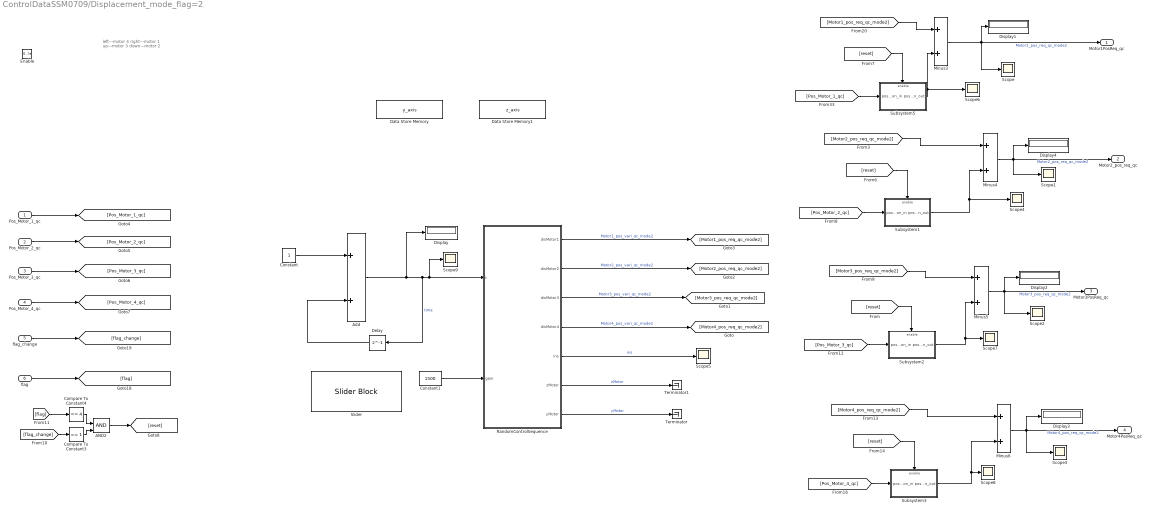
== system ControlDataSSM0709/Displacement_mode_flag=2 ==
  note: left---motor 4
      | right---motor 1
      | up---motor 3
      | down---motor 2
  Pos_Motor_1_qc : Inport
  Pos_Motor_2_qc : Inport  Port=2
  Pos_Motor_3_qc : Inport  Port=3
  Pos_Motor_4_qc : Inport  Port=4
  flag_change : Inport  Port=5
  flag : Inport  Port=6
  Enable : EnablePort  StatesWhenEnabling=reset
  AND2 : Logic  IconShape=distinctive  AllPortsSameDT=off  OutDataTypeStr=boolean
  Add : Sum
  Compare To Constant3 : simulink/Logic and Bit Operations/Compare To Constant  relop===  const=1  OutDataTypeStr=boolean
  Compare To Constant4 : simulink/Logic and Bit Operations/Compare To Constant  relop===  const=4  OutDataTypeStr=boolean
  Constant : Constant
  Constant1 : Constant  Value=1500
  Data Store Memory : DataStoreMemory  DataStoreName=y_axis  WriteAfterWriteMsg=warning  InitialValue=x  ShowAdditionalParam=off  OutDataTypeStr=double
  Data Store Memory1 : DataStoreMemory  DataStoreName=z_axis  WriteAfterWriteMsg=warning  InitialValue=y  ShowAdditionalParam=off  OutDataTypeStr=double
  Delay : Delay  DelayLength=1
  Display{,1..4} (5 alike) : Display
  Minus{3..6} (4 alike) : Sum
  RandomControlSequence : MATLAB Function  TreatAsAtomicUnit=on
  Scope{,1..9} (10 alike) : Scope
  Slider : SliderBlock  ScaleMin=200  ScaleMax=8000
  Subsystem1 : Subsystem
  Subsystem2 : Subsystem
  Subsystem3 : Subsystem
  Subsystem5 : Subsystem
  Terminator : Terminator
  Terminator1 : Terminator
  Motor1PosReq_qc : Outport
  Motor2_pos_req_qc : Outport  Port=2
  Motor3PosReq_qc : Outport  Port=3
  Motor4PosReq_qc : Outport  Port=4
  wires:
  Pos_Motor_4_qc/1 -> [Pos_Motor_4_qc]
  Pos_Motor_3_qc/1 -> [Pos_Motor_3_qc]
  Pos_Motor_2_qc/1 -> [Pos_Motor_2_qc]
  Pos_Motor_1_qc/1 -> [Pos_Motor_1_qc]
  flag/1 -> [flag]
  flag_change/1 -> [flag_change]
  [Pos_Motor_1_qc] -> Subsystem5/1(position_in)
  [reset] -> Subsystem5/Enable
  [Motor1_pos_req_qc_mode2] -> Minus3/1
  Minus3/1 -> Scope/1, Display1/1, Motor1PosReq_qc/1  "Motor1_pos_req_qc_mode2"
  Subsystem5/1(position_out) -> Minus3/2, Scope6/1
  [Motor2_pos_req_qc_mode2] -> Minus4/1
  [reset] -> Subsystem1/Enable
  [Pos_Motor_2_qc] -> Subsystem1/1(position_in)
  Minus4/1 -> Scope1/1, Display4/1, Motor2_pos_req_qc/1  "Motor2_pos_req_qc_mode2"
  Minus5/1 -> Scope2/1, Motor3PosReq_qc/1, Display2/1  "Motor3_pos_req_qc_mode2"
  [reset] -> Subsystem2/Enable
  [Pos_Motor_3_qc] -> Subsystem2/1(position_in)
  [Motor3_pos_req_qc_mode2] -> Minus5/1
  Minus6/1 -> Scope3/1, Motor4PosReq_qc/1, Display3/1  "Motor4_pos_req_qc_mode2"
  [reset] -> Subsystem3/Enable
  [Pos_Motor_4_qc] -> Subsystem3/1(position_in)
  [Motor4_pos_req_qc_mode2] -> Minus6/1
  Compare To Constant4/1 -> AND2/1
  Compare To Constant3/1 -> AND2/2
  [flag_change] -> Compare To Constant3/1
  [flag] -> Compare To Constant4/1
  AND2/1 -> [reset]
  Subsystem2/1(position_out) -> Minus5/2, Scope7/1
  Subsystem3/1(position_out) -> Minus6/2, Scope8/1
  Subsystem1/1(position_out) -> Minus4/2, Scope4/1
  RandomControlSequence/4(disMotor4) -> [Motor4_pos_req_qc_mode2]  "Motor4_pos_vari_qc_mode2"
  RandomControlSequence/3(disMotor3) -> [Motor3_pos_req_qc_mode2]  "Motor3_pos_vari_qc_mode2"
  RandomControlSequence/2(disMotor2) -> [Motor2_pos_req_qc_mode2]  "Motor2_pos_vari_qc_mode2"
  RandomControlSequence/1(disMotor1) -> [Motor1_pos_req_qc_mode2]  "Motor1_pos_vari_qc_mode2"
  Constant/1 -> Add/1
  Add/1 -> Display/1, Delay/1, Scope9/1, RandomControlSequence/1(t)  "time"
  Delay/1 -> Add/2
  RandomControlSequence/5(ins) -> Scope5/1  "ins"
  Constant1/1 -> RandomControlSequence/2(gain)
  RandomControlSequence/7(yMotor) -> Terminator/1  "yMotor"
  RandomControlSequence/6(zMotor) -> Terminator1/1  "zMotor"

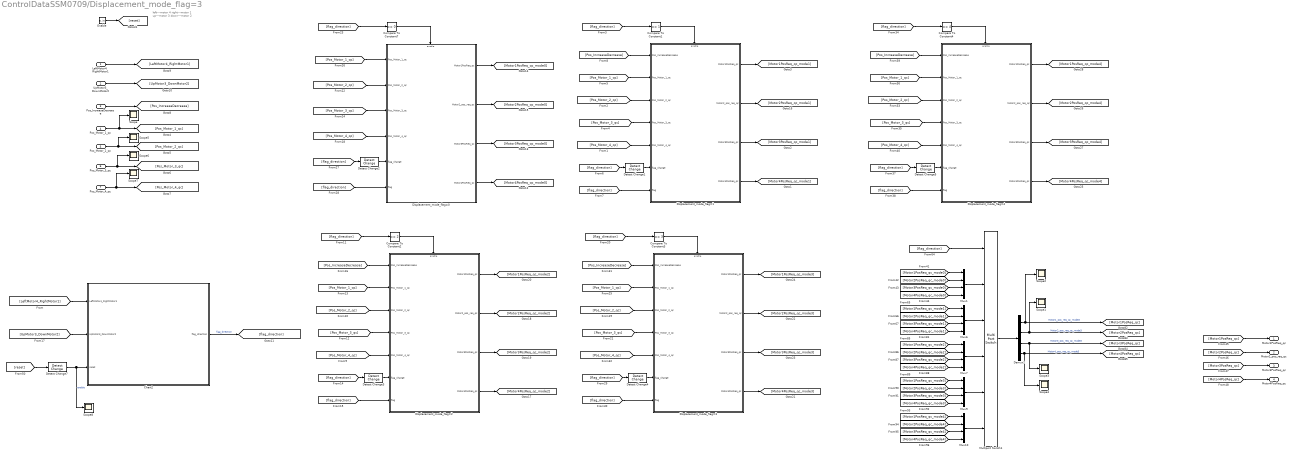
== system ControlDataSSM0709/Displacement_mode_flag=3 ==
  note: left---motor 4
      | right---motor 1
      | up---motor 3
      | down---motor 2
  LeftMotor4_RightMotor1 : Inport
  UpMotor3_DownMotor2 : Inport  Port=2
  Pos_IncreaseDecrease : Inport  Port=3
  Pos_Motor_1_qc : Inport  Port=4
  Pos_Motor_2_qc : Inport  Port=5
  Pos_Motor_3_qc : Inport  Port=6
  Pos_Motor_4_qc : Inport  Port=7
  Enable : EnablePort  StatesWhenEnabling=reset  ShowOutputPort=on
  Chart2 : Stateflow chart  TreatAsAtomicUnit=on
  Compare To Constant1 : simulink/Logic and Bit Operations/Compare To Constant  relop===  const=1  OutDataTypeStr=boolean
  Compare To Constant2 : simulink/Logic and Bit Operations/Compare To Constant  relop===  const=2  OutDataTypeStr=boolean
  Compare To Constant3 : simulink/Logic and Bit Operations/Compare To Constant  relop===  const=3  OutDataTypeStr=boolean
  Compare To Constant4 : simulink/Logic and Bit Operations/Compare To Constant  relop===  const=4  OutDataTypeStr=boolean
  Compare To Constant7 : simulink/Logic and Bit Operations/Compare To Constant  relop===  const=0  OutDataTypeStr=boolean
  Demux2 : Demux
  Detect Change{1..5,7} (6 alike) : simulink/Logic and Bit Operations/Detect Change  vinit=0  OutDataTypeStr=boolean
  Displacement_mode_flag=0 : Subsystem
  Displacement_mode_flag=1 : Subsystem
  Displacement_mode_flag=2 : Subsystem
  Displacement_mode_flag=3 : Subsystem
  Displacement_mode_flag=4 : Subsystem
  Multiport Switch1 : MultiPortSwitch  DataPortOrder=Zero-based contiguous  Inputs=5  zeroidx=on  SaturateOnIntegerOverflow=off  InputSameDT=off
  Mux{1,6..7,9..10} (5 alike) : Mux
  Scope{,1..8} (9 alike) : Scope
  Motor1PosReq_qc : Outport
  Motor2_pos_req_qc : Outport  Port=2
  Motor3PosReq_qc : Outport  Port=3
  Motor4PosReq_qc : Outport  Port=4
  wires:
  LeftMotor4_RightMotor1/1 -> [LeftMotor4_RightMotor1]
  UpMotor3_DownMotor2/1 -> [UpMotor3_DownMotor2]
  Pos_Motor_4_qc/1 -> Scope7/1, [Pos_Motor_4_qc]
  Pos_Motor_3_qc/1 -> Scope6/1, [Pos_Motor_3_qc]
  Pos_Motor_2_qc/1 -> Scope5/1, [Pos_Motor_2_qc]
  Pos_Motor_1_qc/1 -> Scope/1, [Pos_Motor_1_qc]
  Pos_IncreaseDecrease/1 -> [Pos_IncreaseDecrease]
  [LeftMotor4_RightMotor1] -> Chart2/1(LeftMotor4_RightMotor1)
  [UpMotor3_DownMotor2] -> Chart2/2(UpMotor3_DownMotor2)
  Chart2/1(flag_direction) -> [flag_direction]  "flag_direction"
  Compare To Constant7/1 -> Displacement_mode_flag=0/Enable
  [flag_direction] -> Detect Change2/1
  [flag_direction] -> Displacement_mode_flag=0/6(flag)
  [Pos_Motor_2_qc] -> Displacement_mode_flag=0/2(Pos_Motor_2_qc)
  [Pos_Motor_4_qc] -> Displacement_mode_flag=0/4(Pos_Motor_4_qc)
  [Pos_Motor_1_qc] -> Displacement_mode_flag=0/1(Pos_Motor_1_qc)
  [Pos_Motor_3_qc] -> Displacement_mode_flag=0/3(Pos_Motor_3_qc)
  [flag_direction] -> Compare To Constant7/1
  Detect Change2/1 -> Displacement_mode_flag=0/5(flag_change)
  Displacement_mode_flag=0/1(Motor1PosReq_qc) -> [Motor1PosReq_qc_mode0]
  Displacement_mode_flag=0/2(Motor2_pos_req_qc) -> [Motor2PosReq_qc_mode0]
  Displacement_mode_flag=0/3(Motor3PosReq_qc) -> [Motor3PosReq_qc_mode0]
  Displacement_mode_flag=0/4(Motor4PosReq_qc) -> [Motor4PosReq_qc_mode0]
  Detect Change1/1 -> Displacement_mode_flag=1/6(flag_change)
  [flag_direction] -> Compare To Constant1/1
  [flag_direction] -> Displacement_mode_flag=1/7(flag)
  [flag_direction] -> Detect Change1/1
  Displacement_mode_flag=1/1(Motor1PosReq_qc) -> [Motor1PosReq_qc_mode1]
  [Pos_Motor_3_qc] -> Displacement_mode_flag=1/4(Pos_Motor_3_qc)
  Displacement_mode_flag=1/4(Motor4PosReq_qc) -> [Motor4PosReq_qc_mode1]
  [Pos_Motor_2_qc] -> Displacement_mode_flag=1/3(Pos_Motor_2_qc)
  Displacement_mode_flag=1/3(Motor3PosReq_qc) -> [Motor3PosReq_qc_mode1]
  [Pos_Motor_4_qc] -> Displacement_mode_flag=1/5(Pos_Motor_4_qc)
  Displacement_mode_flag=1/2(Motor2_pos_req_qc) -> [Motor2PosReq_qc_mode1]
  Compare To Constant1/1 -> Displacement_mode_flag=1/Enable
  [Pos_IncreaseDecrease] -> Displacement_mode_flag=1/1(Pos_IncreaseDecrease)
  [Pos_Motor_1_qc] -> Displacement_mode_flag=1/2(Pos_Motor_1_qc)
  Demux2/2 -> Scope1/1, [Motor2PosReq_qc]  "Motor2_pos_req_qc_mode3"
  [Motor4PosReq_qc_mode2] -> Mux7/4
  [Motor1PosReq_qc_mode2] -> Mux7/1
  Demux2/3 -> Scope3/1, [Motor3PosReq_qc]  "Motor3_pos_req_qc_mode3"
  [Motor2PosReq_qc_mode2] -> Mux7/2
  [flag_direction] -> Multiport Switch1/1
  Multiport Switch1/1 -> Demux2/1
  [Motor1PosReq_qc_mode1] -> Mux6/1
  [Motor4PosReq_qc_mode4] -> Mux10/4
  [Motor3PosReq_qc_mode1] -> Mux6/3
  [Motor3PosReq_qc_mode2] -> Mux7/3
  Demux2/4 -> Scope4/1, [Motor4PosReq_qc]  "Motor4_pos_req_qc_mode3"
  [Motor3PosReq_qc_mode4] -> Mux10/3
  [Motor2PosReq_qc_mode1] -> Mux6/2
  [Motor3PosReq_qc_mode3] -> Mux9/3
  [Motor4PosReq_qc_mode3] -> Mux9/4
  [Motor4PosReq_qc_mode1] -> Mux6/4
  [Motor2PosReq_qc_mode3] -> Mux9/2
  [Motor2PosReq_qc_mode4] -> Mux10/2
  [Motor1PosReq_qc_mode4] -> Mux10/1
  [Motor1PosReq_qc_mode3] -> Mux9/1
  Demux2/1 -> Scope2/1, [Motor1PosReq_qc]  "Motor1_pos_req_qc_mode3"
  [Pos_Motor_2_qc] -> Displacement_mode_flag=2/3(Pos_Motor_2_qc)
  Compare To Constant2/1 -> Displacement_mode_flag=2/Enable
  Displacement_mode_flag=2/2(Motor2_pos_req_qc) -> [Motor2PosReq_qc_mode2]
  [Pos_Motor_4_qc] -> Displacement_mode_flag=2/5(Pos_Motor_4_qc)
  Displacement_mode_flag=2/4(Motor4PosReq_qc) -> [Motor4PosReq_qc_mode2]
  [Pos_IncreaseDecrease] -> Displacement_mode_flag=2/1(Pos_IncreaseDecrease)
  Displacement_mode_flag=2/3(Motor3PosReq_qc) -> [Motor3PosReq_qc_mode2]
  [flag_direction] -> Compare To Constant2/1
  Displacement_mode_flag=2/1(Motor1PosReq_qc) -> [Motor1PosReq_qc_mode2]
  [Pos_Motor_1_qc] -> Displacement_mode_flag=2/2(Pos_Motor_1_qc)
  [flag_direction] -> Displacement_mode_flag=2/7(flag)
  [flag_direction] -> Detect Change3/1
  [Pos_Motor_3_qc] -> Displacement_mode_flag=2/4(Pos_Motor_3_qc)
  Detect Change3/1 -> Displacement_mode_flag=2/6(flag_change)
  [Pos_Motor_4_qc] -> Displacement_mode_flag=3/5(Pos_Motor_4_qc)
  Displacement_mode_flag=3/2(Motor2_pos_req_qc) -> [Motor2PosReq_qc_mode3]
  Compare To Constant3/1 -> Displacement_mode_flag=3/Enable
  [Pos_Motor_2_qc] -> Displacement_mode_flag=3/3(Pos_Motor_2_qc)
  Displacement_mode_flag=3/4(Motor4PosReq_qc) -> [Motor4PosReq_qc_mode3]
  [Pos_IncreaseDecrease] -> Displacement_mode_flag=3/1(Pos_IncreaseDecrease)
  Detect Change4/1 -> Displacement_mode_flag=3/6(flag_change)
  [flag_direction] -> Displacement_mode_flag=3/7(flag)
  Displacement_mode_flag=3/1(Motor1PosReq_qc) -> [Motor1PosReq_qc_mode3]
  [Pos_Motor_1_qc] -> Displacement_mode_flag=3/2(Pos_Motor_1_qc)
  [flag_direction] -> Compare To Constant3/1
  Displacement_mode_flag=3/3(Motor3PosReq_qc) -> [Motor3PosReq_qc_mode3]
  [Pos_Motor_3_qc] -> Displacement_mode_flag=3/4(Pos_Motor_3_qc)
  [flag_direction] -> Detect Change4/1
  [flag_direction] -> Detect Change5/1
  [Pos_Motor_3_qc] -> Displacement_mode_flag=4/4(Pos_Motor_3_qc)
  Displacement_mode_flag=4/3(Motor3PosReq_qc) -> [Motor3PosReq_qc_mode4]
  [flag_direction] -> Compare To Constant4/1
  [Pos_Motor_1_qc] -> Displacement_mode_flag=4/2(Pos_Motor_1_qc)
  Displacement_mode_flag=4/1(Motor1PosReq_qc) -> [Motor1PosReq_qc_mode4]
  [flag_direction] -> Displacement_mode_flag=4/7(flag)
  Detect Change5/1 -> Displacement_mode_flag=4/6(flag_change)
  [Pos_IncreaseDecrease] -> Displacement_mode_flag=4/1(Pos_IncreaseDecrease)
  Displacement_mode_flag=4/4(Motor4PosReq_qc) -> [Motor4PosReq_qc_mode4]
  [Pos_Motor_2_qc] -> Displacement_mode_flag=4/3(Pos_Motor_2_qc)
  Compare To Constant4/1 -> Displacement_mode_flag=4/Enable
  Displacement_mode_flag=4/2(Motor2_pos_req_qc) -> [Motor2PosReq_qc_mode4]
  [Pos_Motor_4_qc] -> Displacement_mode_flag=4/5(Pos_Motor_4_qc)
  [Motor4PosReq_qc_mode0] -> Mux1/4
  [Motor2PosReq_qc_mode0] -> Mux1/2
  [Motor3PosReq_qc_mode0] -> Mux1/3
  [Motor1PosReq_qc_mode0] -> Mux1/1
  Mux1/1 -> Multiport Switch1/2
  Mux6/1 -> Multiport Switch1/3
  Mux7/1 -> Multiport Switch1/4
  Mux9/1 -> Multiport Switch1/5
  Mux10/1 -> Multiport Switch1/6
  [Motor1PosReq_qc] -> Motor1PosReq_qc/1
  [Motor2PosReq_qc] -> Motor2_pos_req_qc/1
  [Motor3PosReq_qc] -> Motor3PosReq_qc/1
  [Motor4PosReq_qc] -> Motor4PosReq_qc/1
  [reset] -> Detect Change7/1
  Enable/1 -> [reset]
  Detect Change7/1 -> Scope8/1, Chart2/3(reset)  "enable"

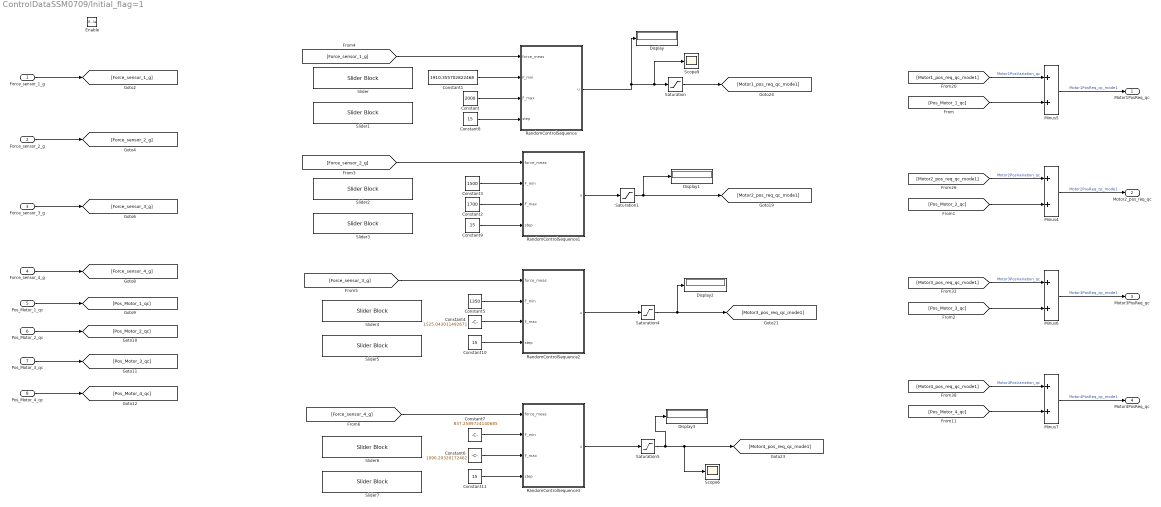
== system ControlDataSSM0709/Initial_flag=1 ==
  Force_sensor_1_g : Inport
  Force_sensor_2_g : Inport  Port=2
  Force_sensor_3_g : Inport  Port=3
  Force_sensor_4_g : Inport  Port=4
  Pos_Motor_1_qc : Inport  Port=5
  Pos_Motor_2_qc : Inport  Port=6
  Pos_Motor_3_qc : Inport  Port=7
  Pos_Motor_4_qc : Inport  Port=8
  Enable : EnablePort
  Constant : Constant  Value=2000
  Constant1 : Constant  Value=1910.355702822468
  Constant{8..11} (4 alike) : Constant  Value=15  SampleTime=0.01
  Constant2 : Constant  Value=1700
  Constant3 : Constant  Value=1500
  Constant4 : Constant  Value=1525.043011492671
  Constant5 : Constant  Value=1350
  Constant6 : Constant  Value=1090.20320172462
  Constant7 : Constant  Value=837.2589724140685
  Display{,1..3} (4 alike) : Display
  Minus{4..7} (4 alike) : Sum
  RandomControlSequence : MATLAB Function  TreatAsAtomicUnit=on
  RandomControlSequence1 : MATLAB Function  TreatAsAtomicUnit=on
  RandomControlSequence2 : MATLAB Function  TreatAsAtomicUnit=on
  RandomControlSequence3 : MATLAB Function  TreatAsAtomicUnit=on
  Saturation{,1,4..5} (4 alike) : Saturate  UpperLimit=200  LowerLimit=-200
  Scope6 : Scope
  Scope9 : Scope
  Slider : SliderBlock  ScaleMin=500  ScaleMax=3000
  Slider1 : SliderBlock  ScaleMin=500  ScaleMax=3000
  Slider2 : SliderBlock  ScaleMin=1000  ScaleMax=3000
  Slider3 : SliderBlock  ScaleMin=1200  ScaleMax=3000
  Slider4 : SliderBlock  ScaleMin=1000  ScaleMax=3000
  Slider5 : SliderBlock  ScaleMin=1200  ScaleMax=3000
  Slider6 : SliderBlock  ScaleMin=500  ScaleMax=2000
  Slider7 : SliderBlock  ScaleMin=500  ScaleMax=2000
  Motor1PosReq_qc : Outport
  Motor2_pos_req_qc : Outport  Port=2
  Motor3PosReq_qc : Outport  Port=3
  Motor4PosReq_qc : Outport  Port=4
  wires:
  [Force_sensor_1_g] -> RandomControlSequence/1(force_meas)
  [Force_sensor_4_g] -> RandomControlSequence3/1(force_meas)
  Saturation/1 -> [Motor1_pos_req_qc_mode1]
  [Force_sensor_3_g] -> RandomControlSequence2/1(force_meas)
  RandomControlSequence/1(u) -> Display/1, Scope9/1, Saturation/1
  Saturation4/1 -> Display2/1, [Motor3_pos_req_qc_mode1]
  Force_sensor_3_g/1 -> [Force_sensor_3_g]
  Force_sensor_4_g/1 -> [Force_sensor_4_g]
  Force_sensor_2_g/1 -> [Force_sensor_2_g]
  Force_sensor_1_g/1 -> [Force_sensor_1_g]
  Saturation1/1 -> [Motor2_pos_req_qc_mode1], Display1/1
  Saturation5/1 -> Display3/1, Scope6/1, [Motor4_pos_req_qc_mode1]
  Pos_Motor_4_qc/1 -> [Pos_Motor_4_qc]
  Pos_Motor_1_qc/1 -> [Pos_Motor_1_qc]
  Pos_Motor_3_qc/1 -> [Pos_Motor_3_qc]
  Pos_Motor_2_qc/1 -> [Pos_Motor_2_qc]
  Minus5/1 -> Motor1PosReq_qc/1  "Motor1PosReq_qc_mode1"
  [Motor1_pos_req_qc_mode1] -> Minus5/1  "Motor1PosVariation_qc"
  [Pos_Motor_1_qc] -> Minus5/2
  Minus4/1 -> Motor2_pos_req_qc/1  "Motor2PosReq_qc_mode1"
  [Motor2_pos_req_qc_mode1] -> Minus4/1  "Motor2PosVariation_qc"
  [Pos_Motor_2_qc] -> Minus4/2
  [Motor3_pos_req_qc_mode1] -> Minus6/1  "Motor3PosVariation_qc"
  Minus6/1 -> Motor3PosReq_qc/1  "Motor3PosReq_qc_mode1"
  [Pos_Motor_3_qc] -> Minus6/2
  [Motor4_pos_req_qc_mode1] -> Minus7/1  "Motor4PosVariation_qc"
  Minus7/1 -> Motor4PosReq_qc/1  "Motor4PosReq_qc_mode1"
  [Pos_Motor_4_qc] -> Minus7/2
  Constant/1 -> RandomControlSequence/3(F_max)
  Constant1/1 -> RandomControlSequence/2(F_min)
  RandomControlSequence1/1(u) -> Saturation1/1
  [Force_sensor_2_g] -> RandomControlSequence1/1(force_meas)
  Constant3/1 -> RandomControlSequence1/2(F_min)
  Constant2/1 -> RandomControlSequence1/3(F_max)
  RandomControlSequence2/1(u) -> Saturation4/1
  Constant4/1 -> RandomControlSequence2/3(F_max)
  Constant5/1 -> RandomControlSequence2/2(F_min)
  RandomControlSequence3/1(u) -> Saturation5/1
  Constant7/1 -> RandomControlSequence3/2(F_min)
  Constant6/1 -> RandomControlSequence3/3(F_max)
  Constant8/1 -> RandomControlSequence/4(step)
  Constant9/1 -> RandomControlSequence1/4(step)
  Constant10/1 -> RandomControlSequence2/4(step)
  Constant11/1 -> RandomControlSequence3/4(step)

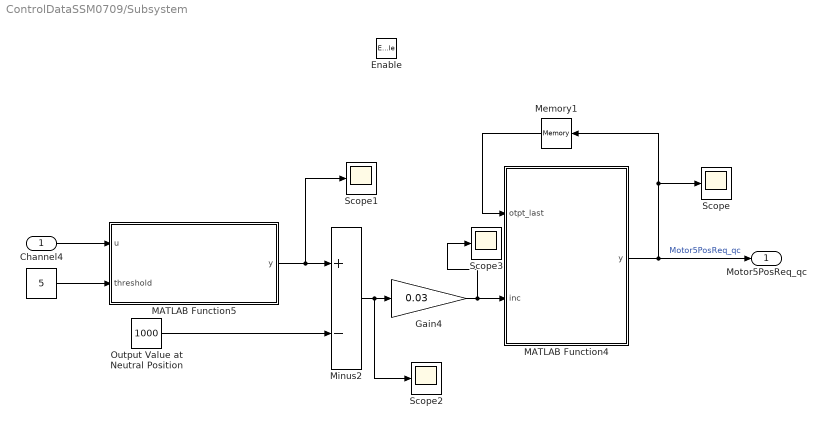
== system ControlDataSSM0709/Subsystem ==
  Channel4 : Inport
  Enable : EnablePort
  " " : Constant  Value=5
  Gain4 : Gain  Gain=0.03
  MATLAB Function4 : MATLAB Function  TreatAsAtomicUnit=on
  MATLAB Function5 : MATLAB Function  TreatAsAtomicUnit=on
  Memory1 : Memory
  Minus2 : Sum  Inputs=+-
  Output Value at Neutral Position : Constant  Value=1000
  Scope{,1..3} (4 alike) : Scope
  Motor5PosReq_qc : Outport
  wires:
  Output Value at Neutral Position/1 -> Minus2/2
  MATLAB Function5/1(y) -> Scope1/1, Minus2/1
  Channel4/1 -> MATLAB Function5/1(u)
  " "/1 -> MATLAB Function5/2(threshold)
  Gain4/1 -> Scope3/1, MATLAB Function4/2(inc)
  Minus2/1 -> Scope2/1, Gain4/1
  Memory1/1 -> MATLAB Function4/1(otpt_last)
  MATLAB Function4/1(y) -> Scope/1, Memory1/1, Motor5PosReq_qc/1  "Motor5PosReq_qc"
